simulink model "lab_02_simulink"  (R2024a)
settings: Solver=VariableStepAuto  StartTime=0.0  StopTime=100  RelTol=1e-3
values from neighbouring files (symbols this model uses):
  b = 4*sqrt(k*m)    [lab_02.m]
  k = 2    [lab_01_gyakorlas.m]    (also in lab_02.m = 150)
  m = 100    [lab_02.m]
libraries: simulink x1
settings Model: Creator=Admin  LastModifiedBy=Admin

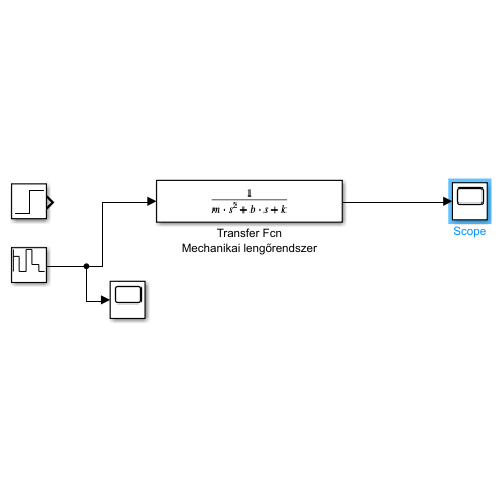
[thumbnail: Simulink's stored preview of the top-level diagram]
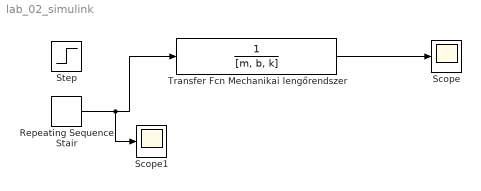
== system lab_02_simulink ==
  Repeating Sequence Stair : simulink/Sources/Repeating Sequence Stair  OutValues=[3 1 4 2 1].'  tsamp=10  OutMin=[]  OutMax=[]  OutDataTypeStr=double  OutputDataTypeScalingMode=double  OutDataType=fixdt(0,8)  ConRadixGroup=Best Precision: Vector-wise  OutScaling=2^-12
  Scope : Scope
  Scope1 : Scope
  Step : Step  SampleTime=0
  Transfer Fcn Mechanikai lengőrendszer : TransferFcn  Denominator=[m, b, k]
  wires:
  Transfer Fcn Mechanikai lengőrendszer/1 -> Scope/1
  Repeating Sequence Stair/1 -> Scope1/1, Transfer Fcn Mechanikai lengőrendszer/1
